simulink library "m3dof_library"  (R2017b)
settings: Solver=ode45  StartTime=0.0  StopTime=10.0  RelTol=1e-3  EnableMultiTasking=on
values from neighbouring files (symbols this model uses):
  l1 = l(1)    [m3dof_jacobian.m]
  l2 = l(2)    [m3dof_jacobian.m]
  l3 = l(3)    [m3dof_jacobian.m]
undefined symbols (not defined in the file or in its folder): eg, I1, I2, I3, m1, m2, m3, mx1, mx2, mx3
settings Model: Creator=Gmalex  LastModifiedBy=david
settings DataIOCC: LimitDataPoints=on  SaveFormat=Array  SignalLoggingSaveFormat=ModelDataLogs
settings OptimizationCC: ExpressionDepthLimit=2147483647  LifeSpan=inf
settings DebuggingCC: UnderspecifiedInitializationDetection=Classic  MergeDetectMultiDrivingBlocksExec=none  SolverPrmCheckMsg=warning  FcnCallInpInsideContextMsg=warning  StateNameClashWarn=warning  SFUnexpectedBacktrackingDiag=warning  SFNoUnconditionalDefaultTransitionDiag=warning  SFExecutionAtInitializationDiag=none
settings HardwareCC: ProdBitPerPointer=32  ProdBitPerSizeT=32  ProdBitPerPtrDiffT=32  ProdLargestAtomicFloat=None  ProdIntDivRoundTo=Undefined  ProdEndianess=Unspecified  ProdWordSize=32  ProdHWDeviceType=32-bit Generic
settings ModelReferenceCC: PropagateSignalLabelsOutOfModel=off
settings CodeAppCC: StateflowObjectComments=on
settings GRTTargetCC: TargetLangStandard=C89/C90 (ANSI)  CombineOutputUpdateFcns=off  GRTInterface=on
settings ConfigComp: CovMetricSettings=dw  CovSaveCumulativeToWorkspaceVar=on  CovSaveSingleToWorkspaceVar=on  CovExternalEMLEnable=off

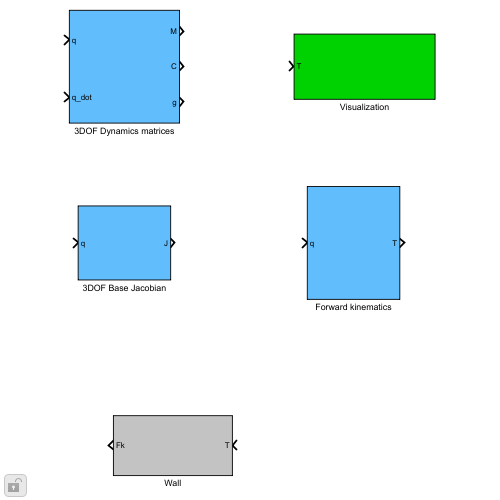
[thumbnail: Simulink's stored preview of the top-level diagram]
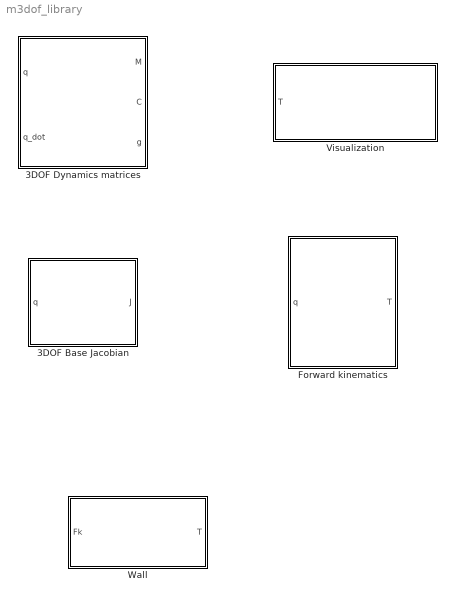
== system m3dof_library ==
  3DOF Base Jacobian : Subsystem  AncestorBlock=library/Forward kinematics  mask{a1=l1, a2=l2, a3=l3}
      mask prompts: a1 "Linklength (Link 1)"; a2 "Linklength (Link 2)"; a3 "Linklength (Link 3)"
      mask help: Base Jacobian of a the 3DoF Manipulator.
  3DOF Dynamics matrices : Subsystem  mask(Dynamics matrices){m1=m1, mX1=mx1, ZZ1=I1, m2=m2, mX2=mx2, ZZ2=I2, m3=m3, mX3=mx3, ZZ3=I3, a1=l1, a2=l2, a3=l3, eg=eg}
      mask prompts: m1 "Mass (Link1)"; mX1 "Massmoment 1. Order (Link1)"; ZZ1 "Massmoment 2. Order (Link 1)"; m2 "Mass (Link2)"; mX2 "Massmoment 1. Order (Link2)"; ZZ2 "Massmoment 2. Order (Link2)"; m3 "Mass (Link3)"; mX3 "Massmoment 1. Order (Link3)"; ZZ3 "Massmoment 2. Order (Link3)"; a1 "Link lenght (Link 1)"; a2 "Link lenght (Link 2)"; a3 "Link lenght (Link 3)"; eg "Gravity direction"
      mask help:
      | Dynamics matrices of the planar 3 Dof manipulator, with q, qdot and eg
      | as joint position, joint velocity and unit vector pointing in (opposite)
      | direction of gravity. The Outputs are M (3x3), C (3x3) and G (3x1) as
      | mass matrix, coriolis and centrifugal matrix and gravity vector.
  Forward kinematics : Subsystem  mask{a1=l1, a2=l2, a3=l3, alpha=0}
      mask prompts: a1 "Linklength (Link 1)"; a2 "Linklength (Link 2)"; a3 "Linklength (Link 3)"; alpha "TCP Orientation"
      mask help:
      | Forward kinematics of the 3DOF planarmanipulator.
      | - q: joint angles
      | - T: bus containing the homogeneous transformation matrices for each link
  Visualization : Subsystem  mask{Ts0=1/16, al=1, a1=l1, a2=l2, a3=l3, alpha=0, eg=eg, tl=50}
      mask prompts: Ts0 "Sample Time Animation"; al "Plot Axis Limit"; a1 "Linklength (Link 1)"; a2 "Linklength (Link 2)"; a3 "Linklength (Link 3)"; alpha "TCP Orientation"; eg "Unitvector (Oposite Gravity direction)"; tl "Tracelength"
      mask help:
      | Visualization utility for the 3DOF planar manipulator.
      | - T: bus containing the homogeneous transformation matrices for each link
  Wall : Subsystem  AncestorBlock=m3dof_library/Wall  mask{x0=[-0.5 0], w=[1 0]}
      mask prompts: x0 "Position of the wall"; w "Orientation of the wall"
      mask help:
      | Cartesian Wall.
      |
      | INPUTS
      | - T: bus containing the homogeneous transformation matrices for each link
      |
      | OUTPUTS
      | - Fk: bus containing the external Cartesian force on each link
      |
      | PARAMETERS
      | - x0: position of the wall (2D)
      | - w: orientation of the wall (2D versor)

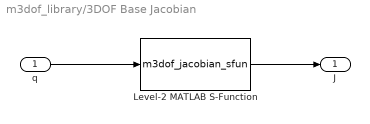
== system m3dof_library/3DOF Base Jacobian ==
  q : Inport
  Level-2 MATLAB S-Function : M-S-Function  FunctionName=m3dof_jacobian_sfun  Parameters=a1,a2,a3
  J : Outport
  wires:
  q/1 -> Level-2 MATLAB S-Function/1
  Level-2 MATLAB S-Function/1 -> J/1

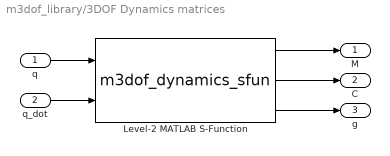
== system m3dof_library/3DOF Dynamics matrices ==
  q : Inport
  q_dot : Inport  Port=2
  Level-2 MATLAB S-Function : M-S-Function  FunctionName=m3dof_dynamics_sfun  Parameters=[m1,mX1,ZZ1],[m2,mX2,ZZ2],[m3,mX3,ZZ3],[a1 a2 a3],-eg
  M : Outport
  C : Outport  Port=2
  g : Outport  Port=3
  wires:
  q/1 -> Level-2 MATLAB S-Function/1
  q_dot/1 -> Level-2 MATLAB S-Function/2
  Level-2 MATLAB S-Function/1 -> M/1
  Level-2 MATLAB S-Function/2 -> C/1
  Level-2 MATLAB S-Function/3 -> g/1

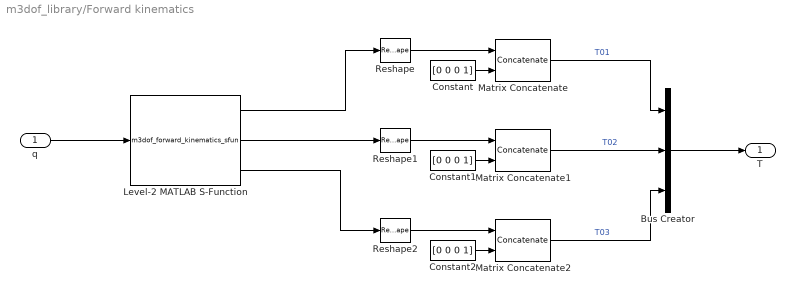
== system m3dof_library/Forward kinematics ==
  q : Inport
  Bus Creator : BusCreator  Inputs=3
  Constant : Constant  Value=[0 0 0 1]  VectorParams1D=off
  Constant1 : Constant  Value=[0 0 0 1]  VectorParams1D=off
  Constant2 : Constant  Value=[0 0 0 1]  VectorParams1D=off
  Level-2 MATLAB S-Function : M-S-Function  FunctionName=m3dof_forward_kinematics_sfun  Parameters=a1,a2,a3
  Matrix Concatenate : Concatenate  Mode=Multidimensional array
  Matrix Concatenate1 : Concatenate  Mode=Multidimensional array
  Matrix Concatenate2 : Concatenate  Mode=Multidimensional array
  Reshape : Reshape  OutputDimensionality=Customize  OutputDimensions=[3,4]
  Reshape1 : Reshape  OutputDimensionality=Customize  OutputDimensions=[3,4]
  Reshape2 : Reshape  OutputDimensionality=Customize  OutputDimensions=[3,4]
  T : Outport
  wires:
  Level-2 MATLAB S-Function/1 -> Reshape/1
  q/1 -> Level-2 MATLAB S-Function/1
  Level-2 MATLAB S-Function/3 -> Reshape2/1
  Level-2 MATLAB S-Function/2 -> Reshape1/1
  Reshape/1 -> Matrix Concatenate/1
  Constant/1 -> Matrix Concatenate/2
  Matrix Concatenate/1 -> Bus Creator/1  "T01"
  Reshape1/1 -> Matrix Concatenate1/1
  Constant1/1 -> Matrix Concatenate1/2
  Constant2/1 -> Matrix Concatenate2/2
  Reshape2/1 -> Matrix Concatenate2/1
  Matrix Concatenate1/1 -> Bus Creator/2  "T02"
  Matrix Concatenate2/1 -> Bus Creator/3  "T03"
  Bus Creator/1 -> T/1

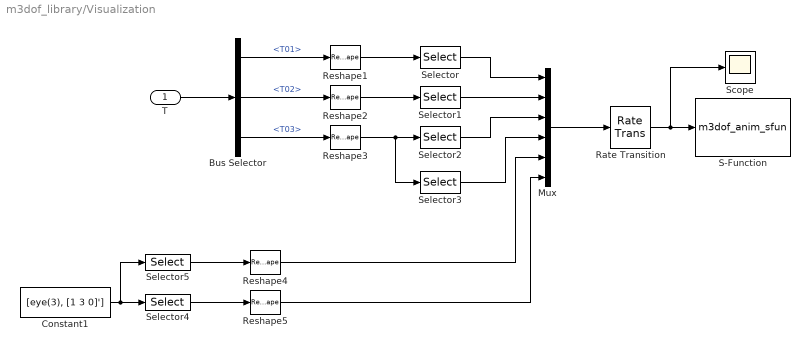
== system m3dof_library/Visualization ==
  T : Inport
  Bus Selector : BusSelector  OutputSignals=T01,T02,T03
  Constant1 : Constant  Value=[eye(3), [1 3 0]']
  Mux : Mux  Inputs=6
  Rate Transition : RateTransition  OutPortSampleTime=Ts0
  Reshape{1..5} (5 alike) : Reshape
  S-Function : S-Function  FunctionName=m3dof_anim_sfun  Parameters=Ts0,al,eg,tl  SFunctionDeploymentMode=off  EnableBusSupport=off
  Scope : Scope
  Selector : Selector  InputPortWidth=16  IndexOptions=Index vector (dialog)  Indices=[13 14]  OutputSizes=1
  Selector1 : Selector  InputPortWidth=16  IndexOptions=Index vector (dialog)  Indices=[13 14]  OutputSizes=1
  Selector2 : Selector  InputPortWidth=16  IndexOptions=Index vector (dialog)  Indices=[13 14]  OutputSizes=1
  Selector3 : Selector  InputPortWidth=16  IndexOptions=Index vector (dialog)  Indices=[1 2 5 6]  OutputSizes=1
  Selector4 : Selector  NumberOfDimensions=2  InputPortWidth=3  IndexOptions=Index vector (dialog),Index vector (dialog)  Indices=1:2,1:2  OutputSizes=1,1
  Selector5 : Selector  NumberOfDimensions=2  InputPortWidth=3  IndexOptions=Index vector (dialog),Index vector (dialog)  Indices=1:2,4  OutputSizes=1,1
  wires:
  Reshape1/1 -> Selector/1
  Reshape2/1 -> Selector1/1
  Reshape3/1 -> Selector2/1, Selector3/1
  Mux/1 -> Rate Transition/1
  Selector/1 -> Mux/1
  Selector1/1 -> Mux/2
  Selector2/1 -> Mux/3
  Rate Transition/1 -> S-Function/1, Scope/1
  Selector3/1 -> Mux/4
  Bus Selector/1 -> Reshape1/1  "<T01>"
  Bus Selector/3 -> Reshape3/1  "<T03>"
  Constant1/1 -> Selector4/1, Selector5/1
  Selector5/1 -> Reshape4/1
  Reshape4/1 -> Mux/5
  Selector4/1 -> Reshape5/1
  Reshape5/1 -> Mux/6
  T/1 -> Bus Selector/1
  Bus Selector/2 -> Reshape2/1  "<T02>"

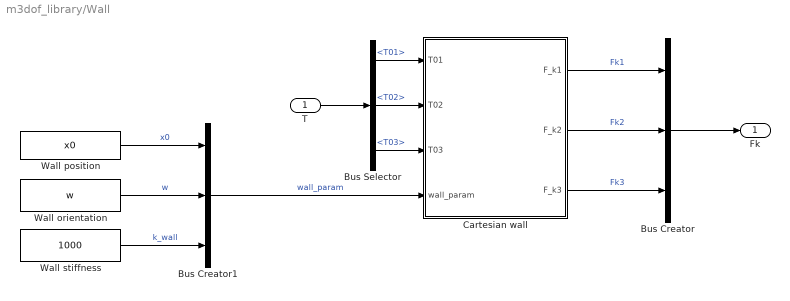
== system m3dof_library/Wall ==
  T : Inport
  Bus Creator : BusCreator  Inputs=3
  Bus Creator1 : BusCreator  Inputs=3
  Bus Selector : BusSelector  OutputSignals=T01,T02,T03
  Cartesian wall : Subsystem
  Wall orientation : Constant  Value=w
  Wall position : Constant  Value=x0
  Wall stiffness : Constant  Value=1000
  Fk : Outport
  wires:
  Bus Creator/1 -> Fk/1
  T/1 -> Bus Selector/1
  Bus Creator1/1 -> Cartesian wall/4(wall_param)  "wall_param"
  Wall position/1 -> Bus Creator1/1  "x0"
  Wall orientation/1 -> Bus Creator1/2  "w"
  Wall stiffness/1 -> Bus Creator1/3  "k_wall"
  Cartesian wall/1(F_k1) -> Bus Creator/1  "Fk1"
  Cartesian wall/2(F_k2) -> Bus Creator/2  "Fk2"
  Cartesian wall/3(F_k3) -> Bus Creator/3  "Fk3"
  Bus Selector/1 -> Cartesian wall/1(T01)  "<T01>"
  Bus Selector/2 -> Cartesian wall/2(T02)  "<T02>"
  Bus Selector/3 -> Cartesian wall/3(T03)  "<T03>"

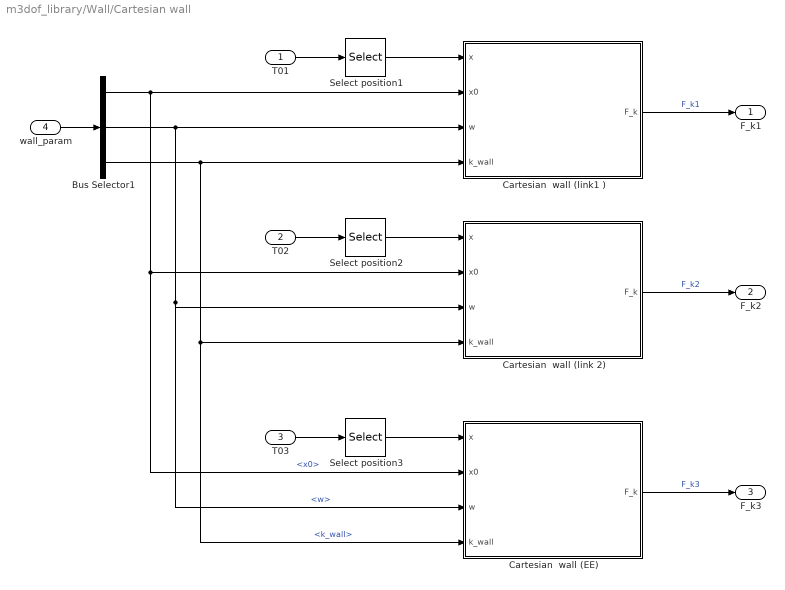
== system m3dof_library/Wall/Cartesian wall ==
  T01 : Inport
  T02 : Inport  Port=2
  T03 : Inport  Port=3
  wall_param : Inport  Port=4
  Bus Selector1 : BusSelector  OutputSignals=x0,w,k_wall
  Cartesian  wall (EE) : MATLAB Function  TreatAsAtomicUnit=on
  Cartesian  wall (link 2) : MATLAB Function  TreatAsAtomicUnit=on
  Cartesian  wall (link1 ) : MATLAB Function  TreatAsAtomicUnit=on
  Select position1 : Selector  NumberOfDimensions=2  InputPortWidth=3  IndexOptions=Index vector (dialog),Index vector (dialog)  Indices=[1 2],4  OutputSizes=1,1
  Select position2 : Selector  NumberOfDimensions=2  InputPortWidth=3  IndexOptions=Index vector (dialog),Index vector (dialog)  Indices=[1 2],4  OutputSizes=1,1
  Select position3 : Selector  NumberOfDimensions=2  InputPortWidth=3  IndexOptions=Index vector (dialog),Index vector (dialog)  Indices=[1 2],4  OutputSizes=1,1
  F_k1 : Outport
  F_k2 : Outport  Port=2
  F_k3 : Outport  Port=3
  wires:
  Select position1/1 -> Cartesian  wall (link1 )/1(x)
  Bus Selector1/1 -> Cartesian  wall (link1 )/2(x0), Cartesian  wall (link 2)/2(x0), Cartesian  wall (EE)/2(x0)  "<x0>"
  Bus Selector1/2 -> Cartesian  wall (link1 )/3(w), Cartesian  wall (link 2)/3(w), Cartesian  wall (EE)/3(w)  "<w>"
  Bus Selector1/3 -> Cartesian  wall (link1 )/4(k_wall), Cartesian  wall (link 2)/4(k_wall), Cartesian  wall (EE)/4(k_wall)  "<k_wall>"
  T01/1 -> Select position1/1
  wall_param/1 -> Bus Selector1/1
  T02/1 -> Select position2/1
  Select position2/1 -> Cartesian  wall (link 2)/1(x)
  T03/1 -> Select position3/1
  Select position3/1 -> Cartesian  wall (EE)/1(x)
  Cartesian  wall (link1 )/1(F_k) -> F_k1/1  "F_k1"
  Cartesian  wall (link 2)/1(F_k) -> F_k2/1  "F_k2"
  Cartesian  wall (EE)/1(F_k) -> F_k3/1  "F_k3"

== matlab function m3dof_library/Wall/Cartesian wall/Cartesian  wall (link1 ) ==
  data: x input; F_k output; x0 input; w input; k_wall input
function F_k = fcn(x,x0,w,k_wall)
% Declaration
F_k = zeros(2,1);

% Normalize direction
w = w/norm(w);

% Distance from the wall
d = w'*(x-x0);

% Reaction of the wall (normal direction)
if(d<0)
    F_k = -k_wall*d*w;
end

== matlab function m3dof_library/Wall/Cartesian wall/Cartesian  wall (link 2) ==
  data: x input; F_k output; x0 input; w input; k_wall input
function F_k = fcn(x,x0,w,k_wall)
% Declaration
F_k = zeros(2,1);

% Normalize direction
w = w/norm(w);

% Distance from the wall
d = w'*(x-x0);

% Reaction of the wall (normal direction)
if(d<0)
    F_k = -k_wall*d*w;
end

== matlab function m3dof_library/Wall/Cartesian wall/Cartesian  wall (EE) ==
  data: x input; F_k output; x0 input; w input; k_wall input
function F_k = fcn(x,x0,w,k_wall)
% Declaration
F_k = zeros(2,1);

% Normalize direction
w = w/norm(w);

% Distance from the wall
d = w'*(x-x0);

% Reaction of the wall (normal direction)
if(d<0)
    F_k = -k_wall*d*w;
end
